simulink model "PID_Ctrl"  (R2019b)
settings: Solver=VariableStepAuto  StartTime=0.0  StopTime=10.0  RelTol=1e-3
settings Model: DataDictionary=Var.sldd  OrderedModelArguments=off  Creator=ip  LastModifiedBy=ip

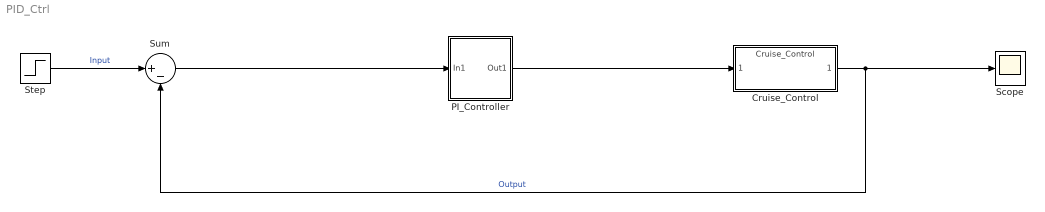
== system PID_Ctrl ==
  Cruise_Control : ModelReference  ModelNameDialog=Cruise_Control  SimulationMode=Normal  ModelReferenceVersion=1.11
  PI_Controller : Subsystem
  Scope : Scope
  Step : Step  Time=0  After=u  SampleTime=0
  Sum : Sum  Inputs=|+-
  wires:
  Cruise_Control/1 -> Sum/2, Scope/1  "Output"
  Step/1 -> Sum/1  "Input"
  Sum/1 -> PI_Controller/1(In1)
  PI_Controller/1(Out1) -> Cruise_Control/1

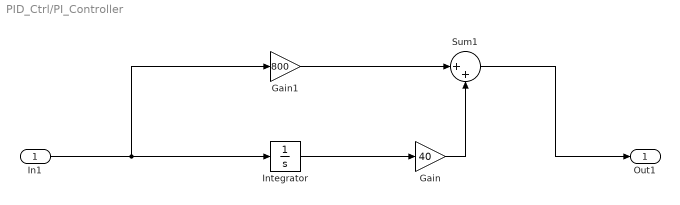
== system PID_Ctrl/PI_Controller ==
  In1 : Inport
  Gain : Gain  Gain=40
  Gain1 : Gain  Gain=800
  Integrator : Integrator
  Sum1 : Sum  Inputs=|++
  Out1 : Outport
  wires:
  Gain1/1 -> Sum1/1
  In1/1 -> Gain1/1, Integrator/1
  Gain/1 -> Sum1/2
  Integrator/1 -> Gain/1
  Sum1/1 -> Out1/1
